simulink model "lab7ex1"  (R2025b)
settings: Solver=ode45  StartTime=0.0  StopTime=Tend  MaxStep=0.001*Ts  MinStep=0.0001*Ts  RelTol=1e-3
values from neighbouring files (symbols this model uses):
  md = MPCInit(Ad,Bd,eye(2),eye(2),zeros(2,1),eye(2),zeros(2,1),Hp,1,1,Hu,1,   		      du_max,du_min,u_max,u_min,[inf inf],   		      [-inf -inf],Q,R,[],[],Ts,0,'qp_as')    [mpc_speedrun.m]
  Ts = 0.05    [mpc_speedrun.m]
libraries: cstblocks x1
settings Model: Creator=davidecovolo  LastModifiedBy=davidecovolo
settings SolverCC: InitialStep=0.0001*Ts

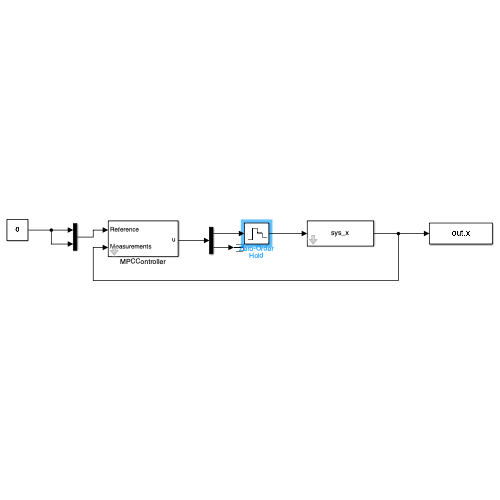
[thumbnail: Simulink's stored preview of the top-level diagram]
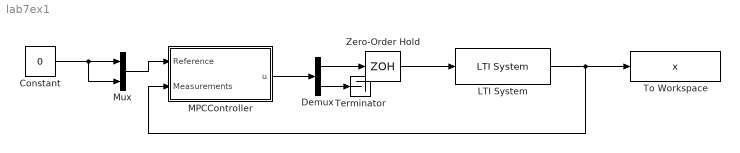
== system lab7ex1 ==
  Constant : Constant  Value=0
  Demux : Demux  Outputs=2
  LTI System : cstblocks/LTI System  sys=sys_x  IC=x0  PadeOrder=0
  MPCController : Subsystem  mask{md=md}
      mask prompts: md "MPCData"
  Mux : Mux  Inputs=2
  Terminator : Terminator
  To Workspace : ToWorkspace  VariableName=x  SaveFormat=Timeseries  SampleTime=-1
  Zero-Order Hold : ZeroOrderHold  SampleTime=Ts
  wires:
  Constant/1 -> Mux/2, Mux/1
  Mux/1 -> MPCController/1(Reference)
  MPCController/1(u) -> Demux/1
  Demux/2 -> Terminator/1
  LTI System/1 -> To Workspace/1, MPCController/2(Measurements)
  Demux/1 -> Zero-Order Hold/1
  Zero-Order Hold/1 -> LTI System/1

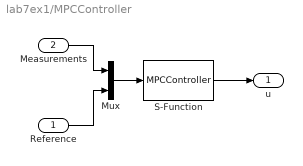
== system lab7ex1/MPCController ==
  Reference : Inport
  Measurements : Inport  Port=2
  Mux : Mux  Inputs=2
  S-Function : S-Function  FunctionName=MPCController  Parameters=md  SFunctionDeploymentMode=off  EnableBusSupport=off
  u : Outport
  wires:
  Mux/1 -> S-Function/1
  Measurements/1 -> Mux/1
  Reference/1 -> Mux/2
  S-Function/1 -> u/1
